simulink model "SIRD_model"  (R2021b)
settings: Solver=FixedStepDiscrete  StartTime=0.0  StopTime=640  FixedStep=1  MaxStep=0.1  RelTol=1e-3
undefined symbols (not defined in the file): DiscIntNeverNeededParam
settings Model: Creator=alex2  LastModifiedBy=alex2

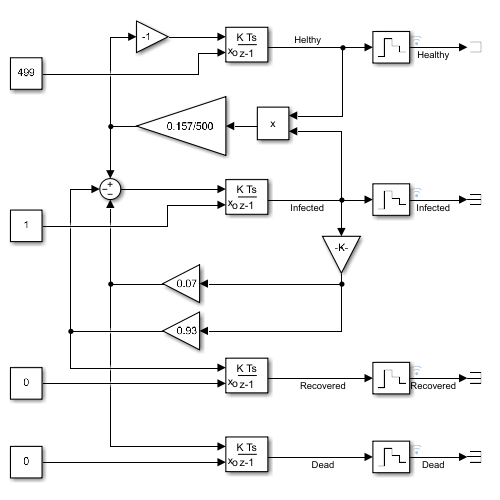
[thumbnail: Simulink's stored preview of the top-level diagram]
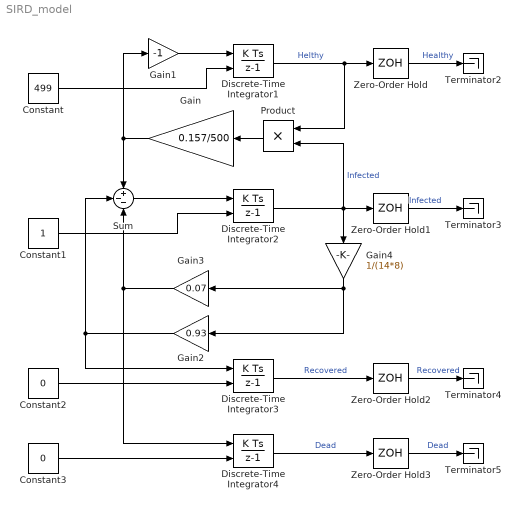
== system SIRD_model ==
  Constant : Constant  Value=499
  Constant1 : Constant
  Constant2 : Constant  Value=0
  Constant3 : Constant  Value=0
  Discrete-Time Integrator{1..4} (4 alike) : DiscreteIntegrator  InitialConditionSource=external  ICPrevOutput=DiscIntNeverNeededParam  ICPrevScaledInput=DiscIntNeverNeededParam
  Gain : Gain  Gain=0.157/500
  Gain1 : Gain  Gain=-1
  Gain2 : Gain  Gain=0.93
  Gain3 : Gain  Gain=0.07
  Gain4 : Gain  Gain=1/(14*8)
  Product : Product
  Sum : Sum  Inputs=+--
  Terminator{2..5} (4 alike) : Terminator
  Zero-Order Hold{,1..3} (4 alike) : ZeroOrderHold  SampleTime=8
  wires:
  Discrete-Time Integrator1/1 -> Zero-Order Hold/1, Product/1  "Helthy"
  Gain/1 -> Gain1/1, Sum/1
  Constant/1 -> Discrete-Time Integrator1/2
  Gain1/1 -> Discrete-Time Integrator1/1
  Product/1 -> Gain/1
  Discrete-Time Integrator2/1 -> Gain4/1, Zero-Order Hold1/1, Product/2  "Infected"
  Constant1/1 -> Discrete-Time Integrator2/2
  Gain2/1 -> Discrete-Time Integrator3/1, Sum/2
  Constant3/1 -> Discrete-Time Integrator4/2
  Constant2/1 -> Discrete-Time Integrator3/2
  Discrete-Time Integrator4/1 -> Zero-Order Hold3/1  "Dead"
  Gain3/1 -> Discrete-Time Integrator4/1, Sum/3
  Discrete-Time Integrator3/1 -> Zero-Order Hold2/1  "Recovered"
  Gain4/1 -> Gain2/1, Gain3/1
  Sum/1 -> Discrete-Time Integrator2/1
  Zero-Order Hold/1 -> Terminator2/1  "Healthy"
  Zero-Order Hold1/1 -> Terminator3/1  "Infected"
  Zero-Order Hold2/1 -> Terminator4/1  "Recovered"
  Zero-Order Hold3/1 -> Terminator5/1  "Dead"
